simulink model "prbs7"  (Simulink 10.1)
settings: Solver=FixedStepDiscrete  StartTime=1  StopTime=127  FixedStep=1  MaxStep=1  RelTol=1e-3  EnableMultiTasking=on
settings Model: Creator=parham  LastModifiedBy=ACER
settings DataIOCC: LimitDataPoints=on  SignalLoggingSaveFormat=ModelDataLogs
settings OptimizationCC: ExpressionDepthLimit=2147483647
settings DebuggingCC: SolverPrmCheckMsg=warning  FcnCallInpInsideContextMsg=warning  StateNameClashWarn=warning

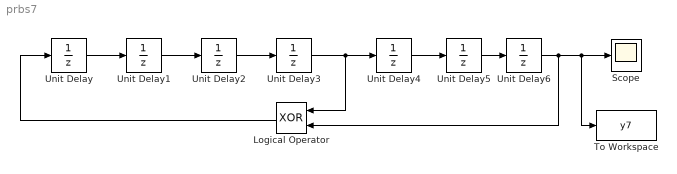
== system prbs7 ==
  Logical Operator : Logic  Operator=XOR  AllPortsSameDT=off  OutDataTypeStr=boolean
  Scope : Scope
  To Workspace : ToWorkspace  VariableName=y7  SampleTime=-1
  Unit Delay{,2,4..6} (5 alike) : UnitDelay  InitialCondition=1  SampleTime=-1  HasFrameUpgradeWarning=on
  Unit Delay1 : UnitDelay  SampleTime=-1  HasFrameUpgradeWarning=on
  Unit Delay3 : UnitDelay  SampleTime=-1  HasFrameUpgradeWarning=on
  wires:
  Unit Delay/1 -> Unit Delay1/1
  Unit Delay3/1 -> Unit Delay4/1, Logical Operator/1
  Unit Delay4/1 -> Unit Delay5/1
  Unit Delay5/1 -> Unit Delay6/1
  Logical Operator/1 -> Unit Delay/1
  Unit Delay1/1 -> Unit Delay2/1
  Unit Delay2/1 -> Unit Delay3/1
  Unit Delay6/1 -> To Workspace/1, Scope/1, Logical Operator/2
